simulink model "FSKSim"  (R2022a)
settings: Solver=VariableStepAuto  StartTime=0.0  StopTime=20.0  RelTol=1e-3
model workspace (MAT data in the model file):
  Width = 1
  f = 1
settings Model: Creator=mluser  LastModifiedBy=mluser
settings DebuggingCC: UnconnectedInputMsg=warning  UnconnectedOutputMsg=warning  UnconnectedLineMsg=warning
settings RTWCC: DLArmComputeVersion=19.05

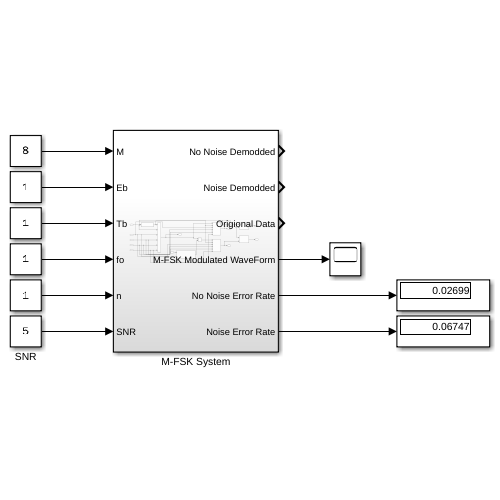
[thumbnail: Simulink's stored preview of the top-level diagram]
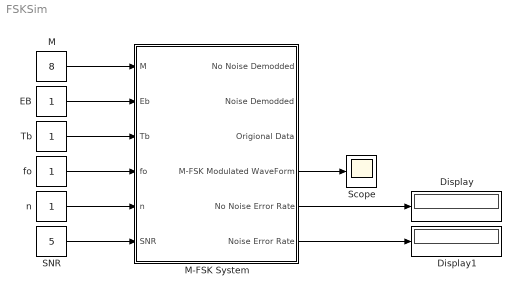
== system FSKSim ==
  Display : Display
  Display1 : Display
  EB : Constant
  M : Constant  Value=8
  M-FSK System : Subsystem
  SNR : Constant  Value=5
  Scope : Scope
  Tb : Constant
  fo : Constant
  n : Constant
  wires:
  M/1 -> M-FSK System/1(M)
  EB/1 -> M-FSK System/2(Eb)
  Tb/1 -> M-FSK System/3(Tb)
  SNR/1 -> M-FSK System/6(SNR)
  fo/1 -> M-FSK System/4(fo)
  n/1 -> M-FSK System/5(n)
  M-FSK System/5(No Noise Error Rate) -> Display/1
  M-FSK System/6(Noise Error Rate) -> Display1/1
  M-FSK System/4(M-FSK Modulated WaveForm) -> Scope/1

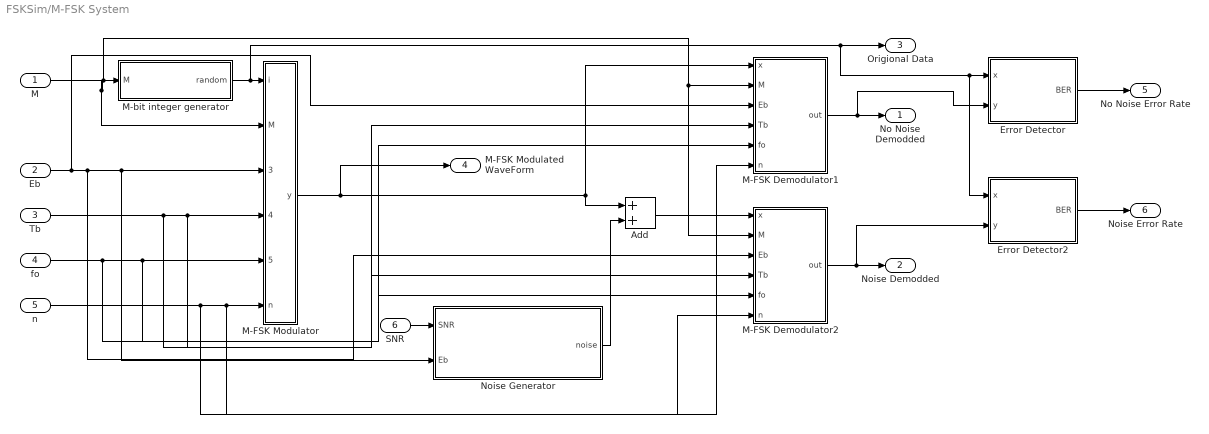
== system FSKSim/M-FSK System ==
  M : Inport
  Eb : Inport  Port=2
  Tb : Inport  Port=3
  fo : Inport  Port=4
  n : Inport  Port=5
  SNR : Inport  Port=6
  Add : Sum
  Error Detector : Subsystem
  Error Detector2 : Subsystem
  M-FSK Demodulator1 : Subsystem
  M-FSK Demodulator2 : Subsystem
  M-FSK Modulator : Subsystem
  M-bit integer generator : Subsystem
  Noise Generator : Subsystem
  No Noise Demodded : Outport
  Noise Demodded : Outport  Port=2
  Origional Data : Outport  Port=3
  M-FSK Modulated WaveForm : Outport  Port=4
  No Noise Error Rate : Outport  Port=5
  Noise Error Rate : Outport  Port=6
  wires:
  Add/1 -> M-FSK Demodulator2/1(x)
  M-FSK Demodulator1/1(out) -> Error Detector/2(y), No Noise Demodded/1
  fo/1 -> M-FSK Demodulator2/5(fo), M-FSK Demodulator1/5(fo), M-FSK Modulator/5(fo)
  SNR/1 -> Noise Generator/1(SNR)
  M-FSK Demodulator2/1(out) -> Error Detector2/2(y), Noise Demodded/1
  M-bit integer generator/1(random) -> Error Detector2/1(x), Error Detector/1(x), Origional Data/1, M-FSK Modulator/1(i)
  M-FSK Modulator/1(y) -> M-FSK Modulated WaveForm/1, M-FSK Demodulator1/1(x), Add/1
  Noise Generator/1(noise) -> Add/2
  Tb/1 -> M-FSK Demodulator1/4(Tb), M-FSK Demodulator2/4(Tb), M-FSK Modulator/4(Tb)
  n/1 -> M-FSK Demodulator2/6(n), M-FSK Demodulator1/6(n), M-FSK Modulator/6(n)
  Eb/1 -> M-FSK Demodulator1/3(Eb), M-FSK Demodulator2/3(Eb), Noise Generator/2(Eb), M-FSK Modulator/3(Eb)
  M/1 -> M-FSK Modulator/2(M), M-FSK Demodulator1/2(M), M-FSK Demodulator2/2(M), M-bit integer generator/1(M)
  Error Detector/1(BER) -> No Noise Error Rate/1
  Error Detector2/1(BER) -> Noise Error Rate/1

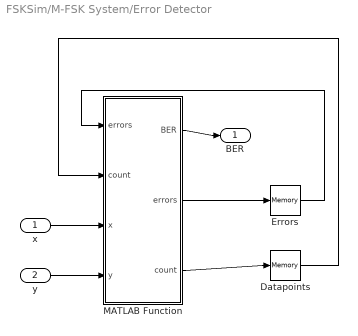
== system FSKSim/M-FSK System/Error Detector ==
  x : Inport
  y : Inport  Port=2
  Datapoints : Memory  InheritSampleTime=on
  Errors : Memory  InheritSampleTime=on
  MATLAB Function : MATLAB Function  TreatAsAtomicUnit=on  SystemSampleTime=0.01
  BER : Outport
  wires:
  MATLAB Function/1(BER) -> BER/1
  MATLAB Function/2(errors) -> Errors/1
  Errors/1 -> MATLAB Function/1("errors ")
  MATLAB Function/3(count) -> Datapoints/1
  Datapoints/1 -> MATLAB Function/2("count ")
  y/1 -> MATLAB Function/4(y)
  x/1 -> MATLAB Function/3(x)

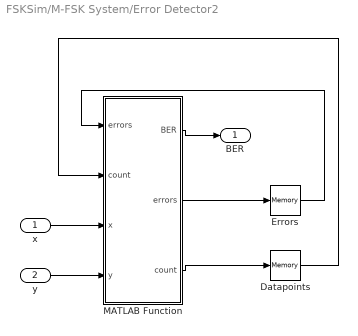
== system FSKSim/M-FSK System/Error Detector2 ==
  x : Inport
  y : Inport  Port=2
  Datapoints : Memory  InheritSampleTime=on
  Errors : Memory  InheritSampleTime=on
  MATLAB Function : MATLAB Function  TreatAsAtomicUnit=on  SystemSampleTime=0.01
  BER : Outport
  wires:
  MATLAB Function/1(BER) -> BER/1
  MATLAB Function/2(errors) -> Errors/1
  Errors/1 -> MATLAB Function/1("errors ")
  MATLAB Function/3(count) -> Datapoints/1
  Datapoints/1 -> MATLAB Function/2("count ")
  y/1 -> MATLAB Function/4(y)
  x/1 -> MATLAB Function/3(x)

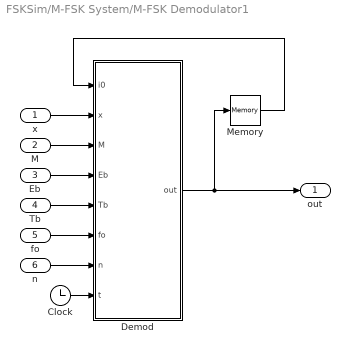
== system FSKSim/M-FSK System/M-FSK Demodulator1 ==
  x : Inport
  M : Inport  Port=2
  Eb : Inport  Port=3
  Tb : Inport  Port=4
  fo : Inport  Port=5
  n : Inport  Port=6
  Clock : Clock
  Demod : MATLAB Function  TreatAsAtomicUnit=on  SystemSampleTime=0.01
  Memory : Memory  InheritSampleTime=on
  out : Outport
  wires:
  Clock/1 -> Demod/8(t)
  x/1 -> Demod/2(x)
  M/1 -> Demod/3(M)
  Eb/1 -> Demod/4(Eb)
  Tb/1 -> Demod/5(Tb)
  fo/1 -> Demod/6(fo)
  n/1 -> Demod/7(n)
  Demod/1(out) -> Memory/1, out/1
  Memory/1 -> Demod/1(i0)

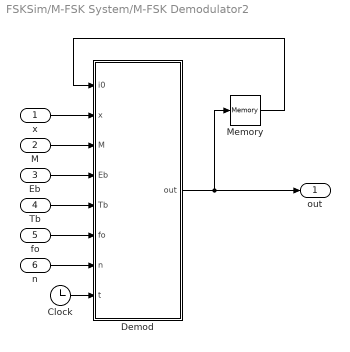
== system FSKSim/M-FSK System/M-FSK Demodulator2 ==
  x : Inport
  M : Inport  Port=2
  Eb : Inport  Port=3
  Tb : Inport  Port=4
  fo : Inport  Port=5
  n : Inport  Port=6
  Clock : Clock
  Demod : MATLAB Function  TreatAsAtomicUnit=on  SystemSampleTime=0.01
  Memory : Memory  InheritSampleTime=on
  out : Outport
  wires:
  Clock/1 -> Demod/8(t)
  x/1 -> Demod/2(x)
  M/1 -> Demod/3(M)
  Eb/1 -> Demod/4(Eb)
  Tb/1 -> Demod/5(Tb)
  fo/1 -> Demod/6(fo)
  n/1 -> Demod/7(n)
  Demod/1(out) -> Memory/1, out/1
  Memory/1 -> Demod/1(i0)

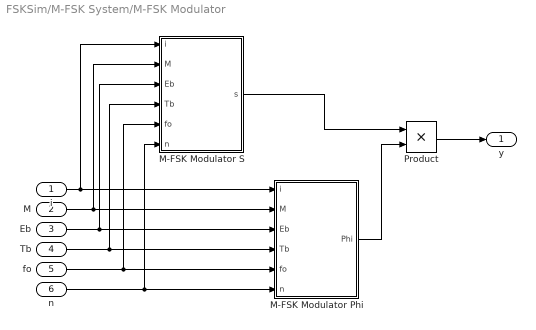
== system FSKSim/M-FSK System/M-FSK Modulator ==
  i : Inport
  M : Inport  Port=2
  Eb : Inport  Port=3
  Tb : Inport  Port=4
  fo : Inport  Port=5
  n : Inport  Port=6
  M-FSK Modulator Phi : Subsystem
  M-FSK Modulator S : Subsystem
  Product : Product
  y : Outport
  wires:
  Tb/1 -> M-FSK Modulator Phi/4(Tb), M-FSK Modulator S/4(Tb)
  M/1 -> M-FSK Modulator Phi/2(M), M-FSK Modulator S/2(M)
  fo/1 -> M-FSK Modulator Phi/5(fo), M-FSK Modulator S/5(fo)
  n/1 -> M-FSK Modulator Phi/6(n), M-FSK Modulator S/6(n)
  i/1 -> M-FSK Modulator Phi/1(i), M-FSK Modulator S/1(i)
  M-FSK Modulator Phi/1(Phi) -> Product/2
  Eb/1 -> M-FSK Modulator Phi/3(Eb), M-FSK Modulator S/3(Eb)
  Product/1 -> y/1
  M-FSK Modulator S/1(s) -> Product/1

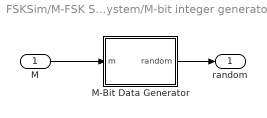
== system FSKSim/M-FSK System/M-bit integer generator ==
  M : Inport
  M-Bit Data Generator : MATLAB Function  TreatAsAtomicUnit=on  SystemSampleTime=2
  random : Outport
  wires:
  M-Bit Data Generator/1(random) -> random/1
  M/1 -> M-Bit Data Generator/1(m)

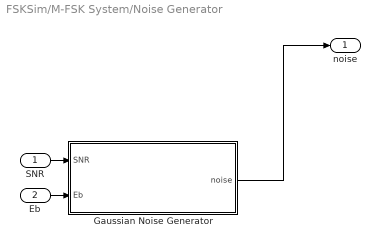
== system FSKSim/M-FSK System/Noise Generator ==
  SNR : Inport
  Eb : Inport  Port=2
  Gaussian Noise Generator : MATLAB Function  TreatAsAtomicUnit=on  SystemSampleTime=0.01
  noise : Outport
  wires:
  Eb/1 -> Gaussian Noise Generator/2(Eb)
  SNR/1 -> Gaussian Noise Generator/1(SNR)
  Gaussian Noise Generator/1(noise) -> noise/1

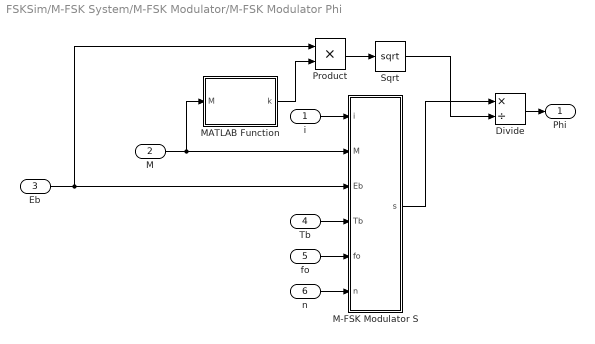
== system FSKSim/M-FSK System/M-FSK Modulator/M-FSK Modulator Phi ==
  i : Inport
  M : Inport  Port=2
  Eb : Inport  Port=3
  Tb : Inport  Port=4
  fo : Inport  Port=5
  n : Inport  Port=6
  Divide : Product  Inputs=*/
  M-FSK Modulator S : Subsystem
  MATLAB Function : MATLAB Function  TreatAsAtomicUnit=on
  Product : Product
  Sqrt : Sqrt
  Phi : Outport
  wires:
  M/1 -> MATLAB Function/1(M), M-FSK Modulator S/2(M)
  i/1 -> M-FSK Modulator S/1(i)
  Eb/1 -> Product/1, M-FSK Modulator S/3(Eb)
  Tb/1 -> M-FSK Modulator S/4(Tb)
  fo/1 -> M-FSK Modulator S/5(fo)
  n/1 -> M-FSK Modulator S/6(n)
  Divide/1 -> Phi/1
  Product/1 -> Sqrt/1
  MATLAB Function/1(k) -> Product/2
  Sqrt/1 -> Divide/2
  M-FSK Modulator S/1(s) -> Divide/1

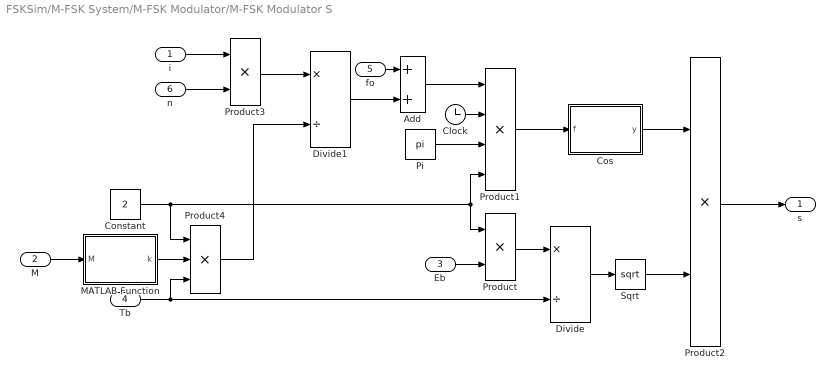
== system FSKSim/M-FSK System/M-FSK Modulator/M-FSK Modulator S ==
  i : Inport
  M : Inport  Port=2
  Eb : Inport  Port=3
  Tb : Inport  Port=4
  fo : Inport  Port=5
  n : Inport  Port=6
  Add : Sum
  Clock : Clock
  Constant : Constant  Value=2
  Cos : MATLAB Function  TreatAsAtomicUnit=on  SystemSampleTime=0.01
  Divide : Product  Inputs=*/
  Divide1 : Product  Inputs=*/
  MATLAB Function : MATLAB Function  TreatAsAtomicUnit=on
  Pi : Constant  Value=pi  OutDataTypeStr=Inherit: Inherit via back propagation
  Product : Product
  Product1 : Product  Inputs=4
  Product2 : Product
  Product3 : Product
  Product4 : Product  Inputs=3
  Sqrt : Sqrt
  s : Outport
  wires:
  Constant/1 -> Product4/1, Product1/4, Product/1
  Eb/1 -> Product/2
  Product/1 -> Divide/1
  Tb/1 -> Product4/3, Divide/2
  Divide/1 -> Sqrt/1
  Pi/1 -> Product1/3
  Clock/1 -> Product1/2
  Product1/1 -> Cos/1(f)
  Sqrt/1 -> Product2/2
  Product2/1 -> s/1
  i/1 -> Product3/1
  n/1 -> Product3/2
  M/1 -> MATLAB Function/1(M)
  MATLAB Function/1(k) -> Product4/2
  Product3/1 -> Divide1/1
  Product4/1 -> Divide1/2
  fo/1 -> Add/1
  Add/1 -> Product1/1
  Divide1/1 -> Add/2
  Cos/1(y) -> Product2/1

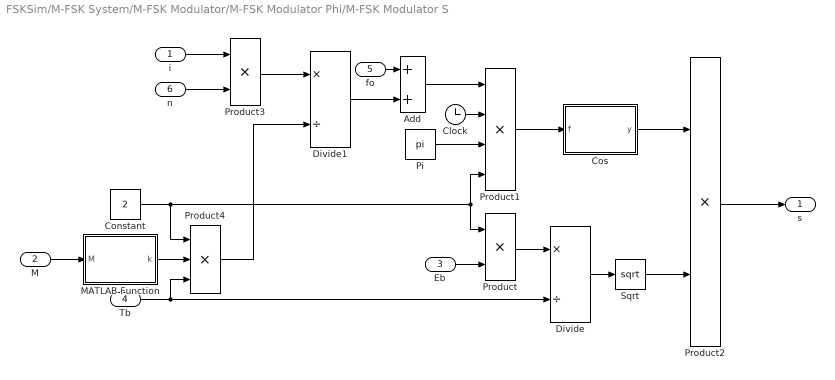
== system FSKSim/M-FSK System/M-FSK Modulator/M-FSK Modulator Phi/M-FSK Modulator S ==
  i : Inport
  M : Inport  Port=2
  Eb : Inport  Port=3
  Tb : Inport  Port=4
  fo : Inport  Port=5
  n : Inport  Port=6
  Add : Sum
  Clock : Clock
  Constant : Constant  Value=2
  Cos : MATLAB Function  TreatAsAtomicUnit=on  SystemSampleTime=0.01
  Divide : Product  Inputs=*/
  Divide1 : Product  Inputs=*/
  MATLAB Function : MATLAB Function  TreatAsAtomicUnit=on
  Pi : Constant  Value=pi  OutDataTypeStr=Inherit: Inherit via back propagation
  Product : Product
  Product1 : Product  Inputs=4
  Product2 : Product
  Product3 : Product
  Product4 : Product  Inputs=3
  Sqrt : Sqrt
  s : Outport
  wires:
  Constant/1 -> Product4/1, Product1/4, Product/1
  Eb/1 -> Product/2
  Product/1 -> Divide/1
  Tb/1 -> Product4/3, Divide/2
  Divide/1 -> Sqrt/1
  Pi/1 -> Product1/3
  Clock/1 -> Product1/2
  Product1/1 -> Cos/1(f)
  Sqrt/1 -> Product2/2
  Product2/1 -> s/1
  i/1 -> Product3/1
  n/1 -> Product3/2
  M/1 -> MATLAB Function/1(M)
  MATLAB Function/1(k) -> Product4/2
  Product3/1 -> Divide1/1
  Product4/1 -> Divide1/2
  fo/1 -> Add/1
  Add/1 -> Product1/1
  Divide1/1 -> Add/2
  Cos/1(y) -> Product2/1

== matlab function FSKSim/M-FSK System/Error Detector2/MATLAB Function ==
  data: errors input; BER output; count input; x input; y input; errors output; count output
function [BER, errors, count] = errorRate(errors, count, x, y)
count = count + 1;
if x ~= y
    errors = errors + 1;
end
BER = errors / count;

== matlab function FSKSim/M-FSK System/M-FSK Modulator/M-FSK Modulator S/Cos ==
  data: f input; y output
function y = cosine(f)

y = cos(f);

== matlab function FSKSim/M-FSK System/M-FSK Modulator/M-FSK Modulator Phi/M-FSK Modulator S/Cos ==
  data: f input; y output
function y = cosine(f)

y = cos(f);

== matlab function FSKSim/M-FSK System/Noise Generator/Gaussian Noise Generator ==
  data: noise output; SNR input; Eb input
function noise = GaussianNoiseGenerator(SNR, Eb)
rng(floor(modposixtime(datetime('now')), 10000));
No = Eb / (10 ^ (SNR / 10));
noise = No * rand * cos(2*pi*rand);

== matlab function FSKSim/M-FSK System/M-bit integer generator/M-Bit Data Generator ==
  data: m input; random output
function random = DataSource(m)
rng(floor(mod(posixtime(datetime('now')), 10000)))
random = randi(m-1);

== matlab function FSKSim/M-FSK System/M-FSK Modulator/M-FSK Modulator S/MATLAB Function ==
  data: M input; k output
function k = logtwo(M)

k = log2(M);

== matlab function FSKSim/M-FSK System/M-FSK Modulator/M-FSK Modulator Phi/M-FSK Modulator S/MATLAB Function ==
  data: M input; k output
function k = logtwo(M)

k = log2(M);

== matlab function FSKSim/M-FSK System/M-FSK Modulator/M-FSK Modulator Phi/MATLAB Function ==
  data: M input; k output
function k = logtwo(M)

k = log2(M);

== matlab function FSKSim/M-FSK System/M-FSK Demodulator2/Demod ==
  data: i0 input; x input; out output; M input; Eb input; Tb input; fo input; n input; t input
function out = demod(i0, x, M, Eb, Tb, fo, n, t)
Best = i0;
s0 = sqrt(2*Eb/Tb)*cos(2*pi*(fo + (i0*n)/(2*Tb*log2(M))));
phi0 = s0/sqrt(Eb*log2(M));
wave0 = s0.*phi0;
Diff = abs(wave0 - x);
for i = 0:1:(M-1)
    s = sqrt(2*Eb/Tb)*cos(2*pi*(fo + (i*n)/(2*Tb*log2(M)))*t);
    phi = s/sqrt(Eb*log2(M));
    wave = s.*phi;
    newDiff = abs(wave - x);
    if newDiff < Diff
        Diff = newDiff;
        Best = i;
    end
end
out = Best;

== matlab function FSKSim/M-FSK System/M-FSK Demodulator1/Demod ==
  data: i0 input; x input; out output; M input; Eb input; Tb input; fo input; n input; t input
function out = demod(i0, x, M, Eb, Tb, fo, n, t)
Best = i0;
s0 = sqrt(2*Eb/Tb)*cos(2*pi*(fo + (i0*n)/(2*Tb*log2(M))));
phi0 = s0/sqrt(Eb*log2(M));
wave0 = s0.*phi0;
Diff = abs(wave0 - x);
for i = 0:1:(M-1)
    s = sqrt(2*Eb/Tb)*cos(2*pi*(fo + (i*n)/(2*Tb*log2(M)))*t);
    phi = s/sqrt(Eb*log2(M));
    wave = s.*phi;
    newDiff = abs(wave - x);
    if newDiff < Diff
        Diff = newDiff;
        Best = i;
    end
end
out = Best;

== matlab function FSKSim/M-FSK System/Error Detector/MATLAB Function ==
  data: errors input; BER output; count input; x input; y input; errors output; count output
function [BER, errors, count] = errorRate(errors, count, x, y)
count = count + 1;
if x ~= y
    errors = errors + 1;
end
BER = errors / count;
